simulink model "Naive_Reduced_Order_Observer"  (R2020a)
settings: Solver=FixedStepAuto  StartTime=0.0  StopTime=10.0  FixedStep=DT  RelTol=1e-3
values from neighbouring files (symbols this model uses):
  L_unknown = 10    [run_Top_Model.m]
  tp = turbine_params_5MW()    [baseline_design.m]    (also in run_Top_Model.m)
undefined symbols (not defined in the file or in its folder): A_pitch, B_pitch, C_pitch, ini_pitch, L_kal_pitch
libraries: simulink x1
settings Model: Creator=lpwoolcock  LastModifiedBy=Vince

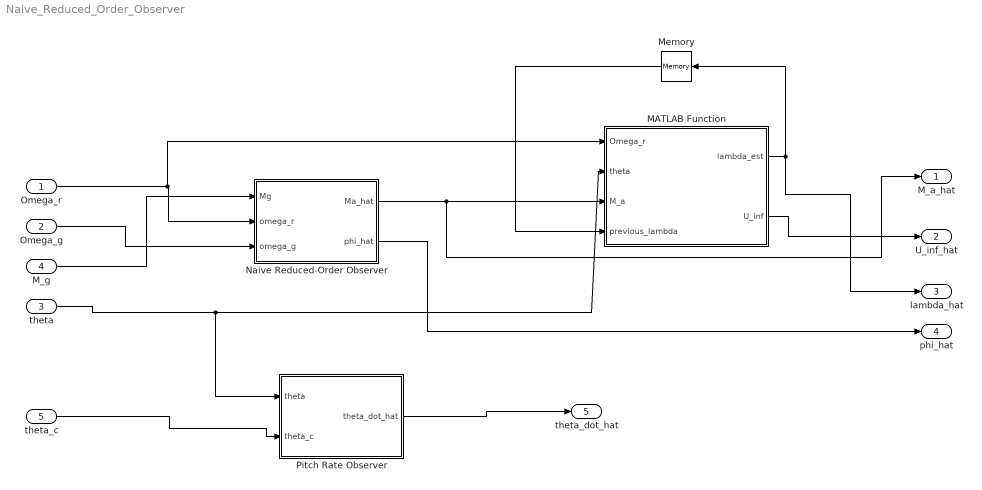
== system Naive_Reduced_Order_Observer ==
  Omega_r : Inport
  Omega_g : Inport  Port=2
  theta : Inport  Port=3
  M_g : Inport  Port=4
  theta_c : Inport  Port=5
  MATLAB Function : MATLAB Function  TreatAsAtomicUnit=on
  Memory : Memory  InitialCondition=tp.lambda_star
  Naive Reduced-Order Observer : Subsystem  TreatAsAtomicUnit=on
  Pitch Rate Observer : Subsystem  TreatAsAtomicUnit=on
  M_a_hat : Outport
  U_inf_hat : Outport  Port=2
  lambda_hat : Outport  Port=3
  phi_hat : Outport  Port=4
  theta_dot_hat : Outport  Port=5
  wires:
  M_g/1 -> Naive Reduced-Order Observer/1(Mg)
  Omega_r/1 -> MATLAB Function/1(Omega_r), Naive Reduced-Order Observer/2(omega_r)
  Omega_g/1 -> Naive Reduced-Order Observer/3(omega_g)
  MATLAB Function/2(U_inf) -> U_inf_hat/1
  MATLAB Function/1(lambda_est) -> Memory/1, lambda_hat/1
  Memory/1 -> MATLAB Function/4(previous_lambda)
  Naive Reduced-Order Observer/1(Ma_hat) -> MATLAB Function/3(M_a), M_a_hat/1
  Naive Reduced-Order Observer/2(phi_hat) -> phi_hat/1
  theta/1 -> Pitch Rate Observer/1(theta), MATLAB Function/2(theta)
  theta_c/1 -> Pitch Rate Observer/2(theta_c)
  Pitch Rate Observer/1(theta_dot_hat) -> theta_dot_hat/1

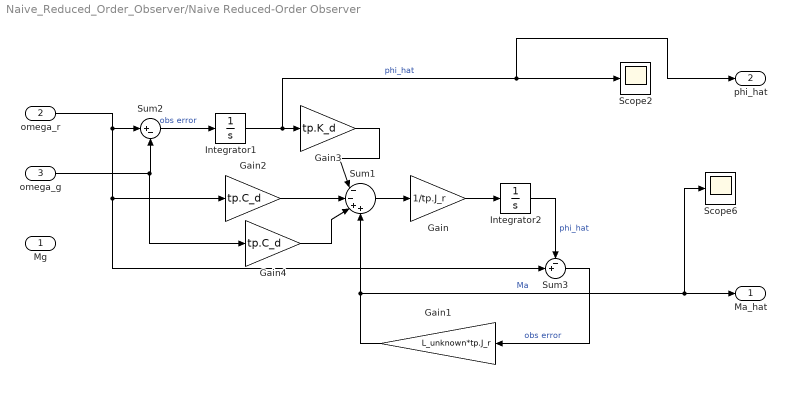
== system Naive_Reduced_Order_Observer/Naive Reduced-Order Observer ==
  Mg : Inport
  omega_r : Inport  Port=2
  omega_g : Inport  Port=3
  Gain : Gain  Gain=1/tp.J_r
  Gain1 : Gain  Gain=L_unknown*tp.J_r
  Gain2 : Gain  Gain=tp.C_d
  Gain3 : Gain  Gain=tp.K_d
  Gain4 : Gain  Gain=tp.C_d
  Integrator1 : Integrator
  Integrator2 : Integrator
  Scope2 : Scope
  Scope6 : Scope
  Sum1 : Sum  Inputs=|--++
  Sum2 : Sum  Inputs=|+-
  Sum3 : Sum  Inputs=-+|
  Ma_hat : Outport
  phi_hat : Outport  Port=2
  wires:
  omega_r/1 -> Gain2/1, Sum3/2, Sum2/1
  omega_g/1 -> Gain4/1, Sum2/2
  Gain1/1 -> Scope6/1, Ma_hat/1, Sum1/4  "Ma"
  Sum2/1 -> Integrator1/1  "obs error"
  Sum1/1 -> Gain/1
  Gain/1 -> Integrator2/1
  Integrator2/1 -> Sum3/1  "phi_hat"
  Sum3/1 -> Gain1/1  "obs error"
  Gain2/1 -> Sum1/2
  Integrator1/1 -> phi_hat/1, Scope2/1, Gain3/1  "phi_hat"
  Gain3/1 -> Sum1/1
  Gain4/1 -> Sum1/3

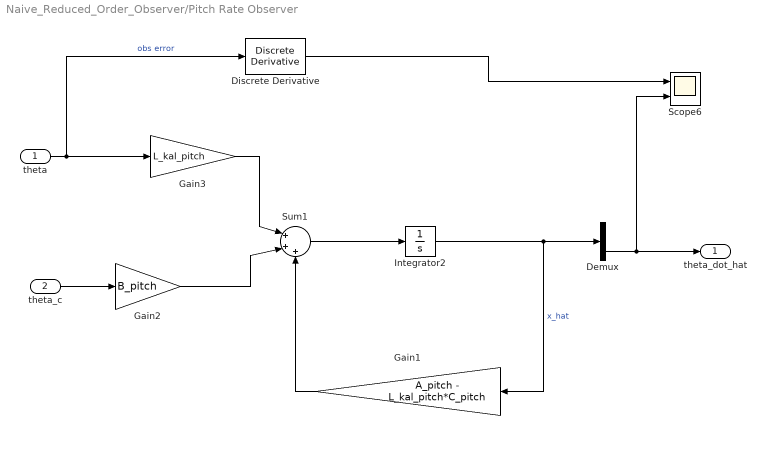
== system Naive_Reduced_Order_Observer/Pitch Rate Observer ==
  theta : Inport
  theta_c : Inport  Port=2
  Demux : Demux  Outputs=2
  Discrete Derivative : simulink/Discrete/Discrete Derivative  gainval=1.0  ICPrevScaledInput=0.0  OutMin=[]  OutMax=[]  OutDataType=fixdt(1, 16)  OutScaling=2^-10  DoSatur=off
  Gain1 : Gain  Gain=A_pitch - L_kal_pitch*C_pitch
  Gain2 : Gain  Gain=B_pitch
  Gain3 : Gain  Gain=L_kal_pitch
  Integrator2 : Integrator  InitialCondition=ini_pitch
  Scope6 : Scope  NumInputPorts=2
  Sum1 : Sum  Inputs=|+++
  theta_dot_hat : Outport
  wires:
  Sum1/1 -> Integrator2/1
  Gain2/1 -> Sum1/2
  Gain3/1 -> Sum1/1
  Integrator2/1 -> Gain1/1, Demux/1  "x_hat"
  theta/1 -> Discrete Derivative/1, Gain3/1  "obs error"
  Gain1/1 -> Sum1/3
  theta_c/1 -> Gain2/1
  Demux/2 -> Scope6/2, theta_dot_hat/1
  Discrete Derivative/1 -> Scope6/1

== matlab function Naive_Reduced_Order_Observer/MATLAB Function ==
  data: Omega_r input; theta input; lambda_est output; M_a input; U_inf output; tp parameter Bus: slBus1; previous_lambda input
% Computes the windspeed using a secant method with given torque
% estimation, rotor speed, and blade pitch angle
function [lambda_est, U_inf] = torque_to_windspeed(Omega_r, theta, M_a, tp, previous_lambda)

% constant in the equation Cp/lambda^3 = C
C = 2*M_a/(tp.rho*pi*(tp.R)^5*(Omega_r)^2);

% Now find the root of f(lambda) = Cp/lambda^3 - C
f = @(lambda) interp2(tp.theta_grid, tp.lambda_grid, tp.C_p, theta, lambda, 'cubic')/(lambda^3) - C;

% Initial guess is previous lambda value
[lambda_est, FVAL, EXITFLAG] = fzero(f, previous_lambda);

% couldn't find valid root, just use optimal lambda for Region 2
if EXITFLAG == -3
    lambda_est = tp.lambda_star; 
end

U_inf = tp.R*Omega_r/lambda_est;

end
